simulink library "LibEEPROM_eeprom_example_ORIGINAL"  (Simulink 10.0)
settings: Solver=VariableStepAuto  StartTime=0.0  StopTime=10.0  RelTol=1e-3
undefined symbols (not defined in the file): CRC32_calc_and_EEPROM_Write_ALL, crc32_calc_intern, CRC32_EEPROM_Read, EEPROM_Mirror, EEPROM_Read, IO_Blk_Lib_TTC500, IO_EEPROM_GetStatus, IO_EEPROM_Init, IO_EEPROM_Write, Read_Mirror, Write_Mirror, Write_Mirror_prepare_EEPROM
libraries: simulink x56
(part 8 of 8)

== system LibEEPROM_eeprom_example_ORIGINAL/EEPROM_WriteRetain/EEPROM_CRC_OK/EEPROM_Mirror ==
  EC_EEPROM_Init : Inport
  EEPROM_Mirror_s : S-Function  FunctionName=EEPROM_Mirror_s  Parameters=SampleTime,offset,length  SFunctionDeploymentMode=off  EnableBusSupport=off
  Terminator : Terminator
  wires:
  EC_EEPROM_Init/1 -> EEPROM_Mirror_s/1
  EEPROM_Mirror_s/1 -> Terminator/1

== system LibEEPROM_eeprom_example_ORIGINAL/EEPROM_WriteRetain/EEPROM_CRC_OK/IO_EEPROM_GetStatus ==
  IO_EEPROM_GetStatus_s : S-Function  FunctionName=IO_EEPROM_GetStatus_s  Parameters=SampleTime  SFunctionDeploymentMode=off  EnableBusSupport=off
  ErrorCode : Outport  VectorParamsAs1DForOutWhenUnconnected=off
  wires:
  IO_EEPROM_GetStatus_s/1 -> ErrorCode/1

== system LibEEPROM_eeprom_example_ORIGINAL/EEPROM_WriteRetain/EEPROM_CRC_OK/IO_EEPROM_GetStatus2 ==
  IO_EEPROM_GetStatus_s : S-Function  FunctionName=IO_EEPROM_GetStatus_s  Parameters=SampleTime  SFunctionDeploymentMode=off  EnableBusSupport=off
  ErrorCode : Outport  VectorParamsAs1DForOutWhenUnconnected=off
  wires:
  IO_EEPROM_GetStatus_s/1 -> ErrorCode/1

== system LibEEPROM_eeprom_example_ORIGINAL/EEPROM_WriteRetain/EEPROM_CRC_OK/IO_EEPROM_Init ==
  IO_EEPROM_Init_s : S-Function  FunctionName=IO_EEPROM_Init_s  Parameters=SampleTime  SFunctionDeploymentMode=off  EnableBusSupport=off
  ErrorCode : Outport  VectorParamsAs1DForOutWhenUnconnected=off
  wires:
  IO_EEPROM_Init_s/1 -> ErrorCode/1

== system LibEEPROM_eeprom_example_ORIGINAL/EEPROM_WriteRetain/EEPROM_CRC_OK/IO_EEPROM_Write_ALL ==
  EC_Write_Mirror : Inport
  GetStatus : Inport  Port=2
  IO_EEPROM_Write_s : S-Function  FunctionName=IO_EEPROM_Write_s  Parameters=SampleTime,offset,length  SFunctionDeploymentMode=off  EnableBusSupport=off
  ErrorCode : Outport  VectorParamsAs1DForOutWhenUnconnected=off
  wires:
  EC_Write_Mirror/1 -> IO_EEPROM_Write_s/1
  GetStatus/1 -> IO_EEPROM_Write_s/2
  IO_EEPROM_Write_s/1 -> ErrorCode/1

== system LibEEPROM_eeprom_example_ORIGINAL/EEPROM_WriteRetain/EEPROM_CRC_OK/Write_Mirror ==
  b_trigger : Inport
  data : Inport  Port=2
  Write_Mirror_s : S-Function  FunctionName=Write_Mirror_s  Parameters=SampleTime,offset,length  SFunctionDeploymentMode=off  EnableBusSupport=off
  ErrorCode_EEPROM_mirror : Outport  VectorParamsAs1DForOutWhenUnconnected=off
  wires:
  b_trigger/1 -> Write_Mirror_s/1
  data/1 -> Write_Mirror_s/2
  Write_Mirror_s/1 -> ErrorCode_EEPROM_mirror/1

== system LibEEPROM_eeprom_example_ORIGINAL/EEPROM_WriteRetain/EEPROM_CRC_OK/crc32_calc_intern ==
  Trigger : TriggerPort  VariantControl=(inherit)
  crc32_calc_intern_s : S-Function  FunctionName=crc32_calc_intern_s  Parameters=SampleTime,EEPROM_mirror,iBasicAddr_intern,iEndAddr_intern  SFunctionDeploymentMode=off  EnableBusSupport=off
  ErrorCode : Outport  VectorParamsAs1DForOutWhenUnconnected=off
  crc32 : Outport  Port=2  VectorParamsAs1DForOutWhenUnconnected=off
  wires:
  crc32_calc_intern_s/2 -> crc32/1
  crc32_calc_intern_s/1 -> ErrorCode/1

== system LibEEPROM_eeprom_example_ORIGINAL/EEPROM_WriteRetain/EEPROM_retain_var_1/Write_Mirror ==
  b_trigger : Inport
  data : Inport  Port=2
  Write_Mirror_s : S-Function  FunctionName=Write_Mirror_s  Parameters=SampleTime,offset,length  SFunctionDeploymentMode=off  EnableBusSupport=off
  ErrorCode_EEPROM_mirror : Outport  VectorParamsAs1DForOutWhenUnconnected=off
  wires:
  Write_Mirror_s/1 -> ErrorCode_EEPROM_mirror/1
  data/1 -> Write_Mirror_s/2
  b_trigger/1 -> Write_Mirror_s/1

== system LibEEPROM_eeprom_example_ORIGINAL/EEPROM_WriteRetain/EEPROM_retain_var_2/Write_Mirror ==
  b_trigger : Inport
  data : Inport  Port=2
  Write_Mirror_s : S-Function  FunctionName=Write_Mirror_s  Parameters=SampleTime,offset,length  SFunctionDeploymentMode=off  EnableBusSupport=off
  ErrorCode_EEPROM_mirror : Outport  VectorParamsAs1DForOutWhenUnconnected=off
  wires:
  Write_Mirror_s/1 -> ErrorCode_EEPROM_mirror/1
  data/1 -> Write_Mirror_s/2
  b_trigger/1 -> Write_Mirror_s/1

== system LibEEPROM_eeprom_example_ORIGINAL/EEPROM_WriteRetain/EEPROM_retain_var_3/Write_Mirror ==
  b_trigger : Inport
  data : Inport  Port=2
  Write_Mirror_s : S-Function  FunctionName=Write_Mirror_s  Parameters=SampleTime,offset,length  SFunctionDeploymentMode=off  EnableBusSupport=off
  ErrorCode_EEPROM_mirror : Outport  VectorParamsAs1DForOutWhenUnconnected=off
  wires:
  Write_Mirror_s/1 -> ErrorCode_EEPROM_mirror/1
  data/1 -> Write_Mirror_s/2
  b_trigger/1 -> Write_Mirror_s/1

== system LibEEPROM_eeprom_example_ORIGINAL/EEPROM_WriteRetain/EEPROM_retain_var_4/Write_Mirror ==
  b_trigger : Inport
  data : Inport  Port=2
  Write_Mirror_s : S-Function  FunctionName=Write_Mirror_s  Parameters=SampleTime,offset,length  SFunctionDeploymentMode=off  EnableBusSupport=off
  ErrorCode_EEPROM_mirror : Outport  VectorParamsAs1DForOutWhenUnconnected=off
  wires:
  Write_Mirror_s/1 -> ErrorCode_EEPROM_mirror/1
  data/1 -> Write_Mirror_s/2
  b_trigger/1 -> Write_Mirror_s/1

== system LibEEPROM_eeprom_example_ORIGINAL/EEPROM_WriteRetain/EEPROM_retain_var_5/Write_Mirror ==
  b_trigger : Inport
  data : Inport  Port=2
  Write_Mirror_s : S-Function  FunctionName=Write_Mirror_s  Parameters=SampleTime,offset,length  SFunctionDeploymentMode=off  EnableBusSupport=off
  ErrorCode_EEPROM_mirror : Outport  VectorParamsAs1DForOutWhenUnconnected=off
  wires:
  Write_Mirror_s/1 -> ErrorCode_EEPROM_mirror/1
  data/1 -> Write_Mirror_s/2
  b_trigger/1 -> Write_Mirror_s/1
